simulink model "k1visetmymon"  (Simulink 8.6)
settings: Solver=VariableStepAuto  StartTime=0.0  StopTime=10.0  RelTol=1e-3
libraries: cdsIPCx x31, cdsFilt x2, cdsAdcx0 x1, cdsAdcx1 x1, cdsAdcx2 x1, VISMON_MASTER x1, cdsModelRate x1, cdsParameters x1
settings Model: Creator=controls  LastModifiedBy=controls
settings DataIOCC: SaveFormat=Dataset  SignalLoggingSaveFormat=Dataset
settings OptimizationCC: ExpressionDepthLimit=128
settings DebuggingCC: UnderspecifiedInitializationDetection=Simplified  MergeDetectMultiDrivingBlocksExec=error  SolverPrmCheckMsg=none  FcnCallInpInsideContextMsg=EnableAllAsError  StateNameClashWarn=none
settings HardwareCC: ProdBitPerPointer=64  ProdLargestAtomicFloat=Float  ProdIntDivRoundTo=Zero  ProdEndianess=LittleEndian  ProdWordSize=64  ProdHWDeviceType=Intel->x86-64 (Windows64)
settings GRTTargetCC: GeneratePreprocessorConditionals=Use local settings  CombineOutputUpdateFcns=on  GRTInterface=off
settings ConfigComp: CovModelRefEnable=off

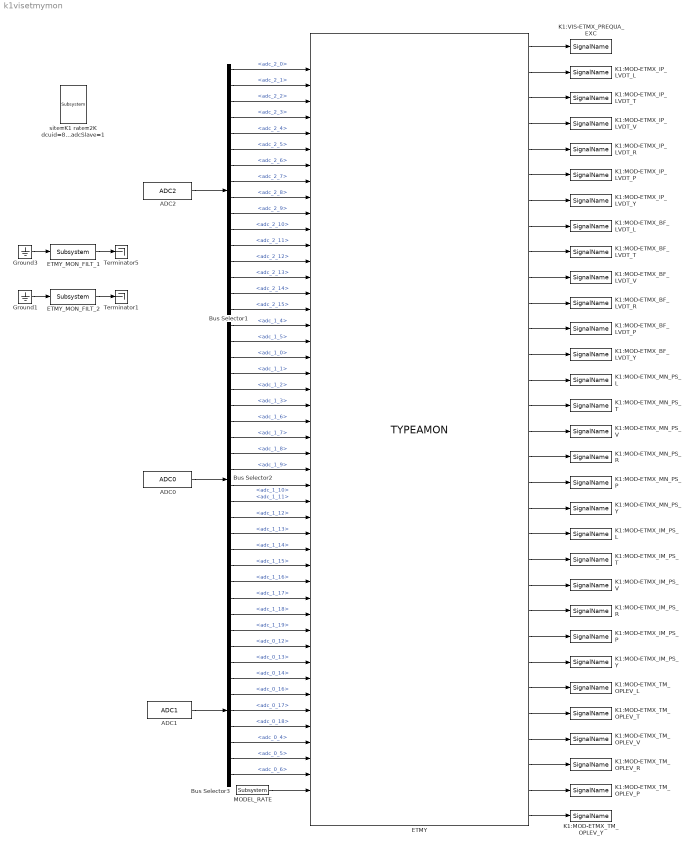
== system k1visetmymon ==
  ADC0 : cdsAdcx0/ADC0  Tag=cdsAdc  Description=|
      | type-GSC_16AI64SSA
      | card_num=0
      settings: AttributesFormatString=%<Description>\n%<Tag>
  ADC1 : cdsAdcx1/ADC1  Tag=cdsAdc  Description=|
      | type-GSC_16AI64SSA
      | card_num=1
      settings: AttributesFormatString=%<Description>\n%<Tag>
  ADC2 : cdsAdcx2/ADC2  Tag=cdsAdc  Description=|
      | type-GSC_16AI64SSA
      | card_num=2
      settings: AttributesFormatString=%<Description>\n%<Tag>
  Bus Selector1 : BusSelector  Description=ADC Selector  OutputSignals=adc_2_0,adc_2_1,adc_2_2,adc_2_3,adc_2_4,adc_2_5,adc_2_6,adc_2_7,adc_2_8,adc_2_9,adc_2_10,adc_2_11,adc_2_12,adc_2_13,adc_2_14,adc_2_15
      settings: AttributesFormatString=%<Description>
  Bus Selector2 : BusSelector  OutputSignals=adc_1_4,adc_1_5,adc_1_0,adc_1_1,adc_1_2,adc_1_3,adc_1_6,adc_1_7,adc_1_8,adc_1_9,adc_1_10,adc_1_11,adc_1_12,adc_1_13,adc_1_14,adc_1_15,adc_1_16,adc_1_17,adc_1_18,adc_1_19
  Bus Selector3 : BusSelector  OutputSignals=adc_0_12,adc_0_13,adc_0_14,adc_0_16,adc_0_17,adc_0_18,adc_0_4,adc_0_5,adc_0_6
  ETMY : VISMON_MASTER/TYPEAMON
  ETMY_MON_FILT_1 : cdsFilt/Subsystem  Tag=cdsFilt  Description=|
      | Purpose:                                                                                                                                                                                                                                  
      | Standard CDS IIR filter module.                                                                                                                                                                                                           
      |                                                                                                                                                                                                                                           
      | Operation:                                                                                                                                                                                                                                
      | Consists of 10 second order section IIR filters, plus a ramped gain stage. In FE code, also provides pre-defined test points and excitation channel inputs. The filter coefficients are defined in the LIGO system using the 'foton' tool.
      |                                                                                                                                                                                                                                           
      | Usage:                                                                                                                                                                                                                                    
      | Name the part with the desired filter module name.
      settings: AttributesFormatString=%<Tag>
  ETMY_MON_FILT_2 : cdsFilt/Subsystem  Tag=cdsFilt  Description=|
      | Purpose:                                                                                                                                                                                                                                  
      | Standard CDS IIR filter module.                                                                                                                                                                                                           
      |                                                                                                                                                                                                                                           
      | Operation:                                                                                                                                                                                                                                
      | Consists of 10 second order section IIR filters, plus a ramped gain stage. In FE code, also provides pre-defined test points and excitation channel inputs. The filter coefficients are defined in the LIGO system using the 'foton' tool.
      |                                                                                                                                                                                                                                           
      | Usage:                                                                                                                                                                                                                                    
      | Name the part with the desired filter module name.
      settings: AttributesFormatString=%<Tag>
  Ground1 : Ground
  Ground3 : Ground
  K1:MOD-ETMX_BF_LVDT_L : cdsIPCx/SignalName  Tag=cdsIPCx_SHMEM  Description=Inter-Process Communication via Shared memory.
      settings: AttributesFormatString=%<Tag>
  K1:MOD-ETMX_BF_LVDT_P : cdsIPCx/SignalName  Tag=cdsIPCx_SHMEM  Description=Inter-Process Communication via Shared memory.
      settings: AttributesFormatString=%<Tag>
  K1:MOD-ETMX_BF_LVDT_R : cdsIPCx/SignalName  Tag=cdsIPCx_SHMEM  Description=Inter-Process Communication via Shared memory.
      settings: AttributesFormatString=%<Tag>
  K1:MOD-ETMX_BF_LVDT_T : cdsIPCx/SignalName  Tag=cdsIPCx_SHMEM  Description=Inter-Process Communication via Shared memory.
      settings: AttributesFormatString=%<Tag>
  K1:MOD-ETMX_BF_LVDT_V : cdsIPCx/SignalName  Tag=cdsIPCx_SHMEM  Description=Inter-Process Communication via Shared memory.
      settings: AttributesFormatString=%<Tag>
  K1:MOD-ETMX_BF_LVDT_Y : cdsIPCx/SignalName  Tag=cdsIPCx_SHMEM  Description=Inter-Process Communication via Shared memory.
      settings: AttributesFormatString=%<Tag>
  K1:MOD-ETMX_IM_PS_L : cdsIPCx/SignalName  Tag=cdsIPCx_SHMEM  Description=Inter-Process Communication via Shared memory.
      settings: AttributesFormatString=%<Tag>
  K1:MOD-ETMX_IM_PS_P : cdsIPCx/SignalName  Tag=cdsIPCx_SHMEM  Description=Inter-Process Communication via Shared memory.
      settings: AttributesFormatString=%<Tag>
  K1:MOD-ETMX_IM_PS_R : cdsIPCx/SignalName  Tag=cdsIPCx_SHMEM  Description=Inter-Process Communication via Shared memory.
      settings: AttributesFormatString=%<Tag>
  K1:MOD-ETMX_IM_PS_T : cdsIPCx/SignalName  Tag=cdsIPCx_SHMEM  Description=Inter-Process Communication via Shared memory.
      settings: AttributesFormatString=%<Tag>
  K1:MOD-ETMX_IM_PS_V : cdsIPCx/SignalName  Tag=cdsIPCx_SHMEM  Description=Inter-Process Communication via Shared memory.
      settings: AttributesFormatString=%<Tag>
  K1:MOD-ETMX_IM_PS_Y : cdsIPCx/SignalName  Tag=cdsIPCx_SHMEM  Description=Inter-Process Communication via Shared memory.
      settings: AttributesFormatString=%<Tag>
  K1:MOD-ETMX_IP_LVDT_L : cdsIPCx/SignalName  Tag=cdsIPCx_SHMEM  Description=Inter-Process Communication via Shared memory.
      settings: AttributesFormatString=%<Tag>
  K1:MOD-ETMX_IP_LVDT_P : cdsIPCx/SignalName  Tag=cdsIPCx_SHMEM  Description=Inter-Process Communication via Shared memory.
      settings: AttributesFormatString=%<Tag>
  K1:MOD-ETMX_IP_LVDT_R : cdsIPCx/SignalName  Tag=cdsIPCx_SHMEM  Description=Inter-Process Communication via Shared memory.
      settings: AttributesFormatString=%<Tag>
  K1:MOD-ETMX_IP_LVDT_T : cdsIPCx/SignalName  Tag=cdsIPCx_SHMEM  Description=Inter-Process Communication via Shared memory.
      settings: AttributesFormatString=%<Tag>
  K1:MOD-ETMX_IP_LVDT_V : cdsIPCx/SignalName  Tag=cdsIPCx_SHMEM  Description=Inter-Process Communication via Shared memory.
      settings: AttributesFormatString=%<Tag>
  K1:MOD-ETMX_IP_LVDT_Y : cdsIPCx/SignalName  Tag=cdsIPCx_SHMEM  Description=Inter-Process Communication via Shared memory.
      settings: AttributesFormatString=%<Tag>
  K1:MOD-ETMX_MN_PS_L : cdsIPCx/SignalName  Tag=cdsIPCx_SHMEM  Description=Inter-Process Communication via Shared memory.
      settings: AttributesFormatString=%<Tag>
  K1:MOD-ETMX_MN_PS_P : cdsIPCx/SignalName  Tag=cdsIPCx_SHMEM  Description=Inter-Process Communication via Shared memory.
      settings: AttributesFormatString=%<Tag>
  K1:MOD-ETMX_MN_PS_R : cdsIPCx/SignalName  Tag=cdsIPCx_SHMEM  Description=Inter-Process Communication via Shared memory.
      settings: AttributesFormatString=%<Tag>
  K1:MOD-ETMX_MN_PS_T : cdsIPCx/SignalName  Tag=cdsIPCx_SHMEM  Description=Inter-Process Communication via Shared memory.
      settings: AttributesFormatString=%<Tag>
  K1:MOD-ETMX_MN_PS_V : cdsIPCx/SignalName  Tag=cdsIPCx_SHMEM  Description=Inter-Process Communication via Shared memory.
      settings: AttributesFormatString=%<Tag>
  K1:MOD-ETMX_MN_PS_Y : cdsIPCx/SignalName  Tag=cdsIPCx_SHMEM  Description=Inter-Process Communication via Shared memory.
      settings: AttributesFormatString=%<Tag>
  K1:MOD-ETMX_TM_OPLEV_L : cdsIPCx/SignalName  Tag=cdsIPCx_SHMEM  Description=Inter-Process Communication via Shared memory.
      settings: AttributesFormatString=%<Tag>
  K1:MOD-ETMX_TM_OPLEV_P : cdsIPCx/SignalName  Tag=cdsIPCx_SHMEM  Description=Inter-Process Communication via Shared memory.
      settings: AttributesFormatString=%<Tag>
  K1:MOD-ETMX_TM_OPLEV_R : cdsIPCx/SignalName  Tag=cdsIPCx_SHMEM  Description=Inter-Process Communication via Shared memory.
      settings: AttributesFormatString=%<Tag>
  K1:MOD-ETMX_TM_OPLEV_T : cdsIPCx/SignalName  Tag=cdsIPCx_SHMEM  Description=Inter-Process Communication via Shared memory.
      settings: AttributesFormatString=%<Tag>
  K1:MOD-ETMX_TM_OPLEV_V : cdsIPCx/SignalName  Tag=cdsIPCx_SHMEM  Description=Inter-Process Communication via Shared memory.
      settings: AttributesFormatString=%<Tag>
  K1:MOD-ETMX_TM_OPLEV_Y : cdsIPCx/SignalName  Tag=cdsIPCx_SHMEM  Description=Inter-Process Communication via Shared memory.
      settings: AttributesFormatString=%<Tag>
  K1:VIS-ETMX_PREQUA_EXC : cdsIPCx/SignalName  Tag=cdsIPCx_SHMEM  Description=Inter-Process Communication via Shared memory.
      settings: AttributesFormatString=%<Tag>
  MODEL_RATE : cdsModelRate/Subsystem  Tag=cdsModelRate
      settings: AttributesFormatString=%<Tag>
  Terminator1 : Terminator
  Terminator5 : Terminator
  site=K1 rate=2K dcuid=80 host=k1ey1 specific_cpu=1 adcSlave=1 : cdsParameters/Subsystem  Tag=cdsParameters  Description=|
      | Purpose:                                                                                                                                                                                                                                
      | Provide system parameters to the FE code generator to properly configure the generated EPICS names, rep rate of the FE controller, and the Data Acquisition node ID for proper storage of data from this FE controller.                 
      |                                                                                                                                                                                                                                         
      | Useage:                                                                                                                                                                                                                                 
      | The part NAME field is used to identify the FE parameters. It must be of the form:                                                                                                                                                      
      | site=                                                                                                                                                                                                                                   
      | rate=                                                                                                                                                                                                                                   
      | dcuid=                                                                                                                                                                                                                                  
      |                                                                                                                                                                                                                                         
      | Where:                                                                                                                                                                                                                                  
      | site= argument may be H1, H2, L1, M1, G1, either as a single argument or multiple, for example site=H1,H2. These are the only names allowed. These will become the first two characters of all EPICS and signal names (for example G1:).
      |                                                                                                                                                                                                                                         
      | rate= may be 2K, 16K, 32K, or 64K                                                                                                                                                                                                       
      |                                                                                                                                                                                                                                         
      | dcuid= is site specific ie it must be unique at each site.
      settings: AttributesFormatString=%<Tag>
  wires:
  ADC2/1 -> Bus Selector1/1
  Ground3/1 -> ETMY_MON_FILT_1/1
  Ground1/1 -> ETMY_MON_FILT_2/1
  ETMY_MON_FILT_1/1 -> Terminator5/1
  ETMY_MON_FILT_2/1 -> Terminator1/1
  Bus Selector1/1 -> ETMY/1  "<adc_2_0>"
  Bus Selector1/2 -> ETMY/2  "<adc_2_1>"
  Bus Selector1/3 -> ETMY/3  "<adc_2_2>"
  Bus Selector1/4 -> ETMY/4  "<adc_2_3>"
  Bus Selector1/5 -> ETMY/5  "<adc_2_4>"
  Bus Selector1/6 -> ETMY/6  "<adc_2_5>"
  Bus Selector1/7 -> ETMY/7  "<adc_2_6>"
  Bus Selector1/8 -> ETMY/8  "<adc_2_7>"
  Bus Selector1/9 -> ETMY/9  "<adc_2_8>"
  Bus Selector1/10 -> ETMY/10  "<adc_2_9>"
  Bus Selector1/11 -> ETMY/11  "<adc_2_10>"
  Bus Selector1/12 -> ETMY/12  "<adc_2_11>"
  Bus Selector1/13 -> ETMY/13  "<adc_2_12>"
  Bus Selector1/14 -> ETMY/14  "<adc_2_13>"
  Bus Selector1/15 -> ETMY/15  "<adc_2_14>"
  Bus Selector1/16 -> ETMY/16  "<adc_2_15>"
  Bus Selector2/2 -> ETMY/18  "<adc_1_5>"
  Bus Selector2/9 -> ETMY/25  "<adc_1_8>"
  Bus Selector2/3 -> ETMY/19  "<adc_1_0>"
  Bus Selector2/8 -> ETMY/24  "<adc_1_7>"
  Bus Selector2/13 -> ETMY/29  "<adc_1_12>"
  Bus Selector2/5 -> ETMY/21  "<adc_1_2>"
  Bus Selector2/14 -> ETMY/30  "<adc_1_13>"
  Bus Selector2/17 -> ETMY/33  "<adc_1_16>"
  Bus Selector2/12 -> ETMY/28  "<adc_1_11>"
  Bus Selector2/16 -> ETMY/32  "<adc_1_15>"
  Bus Selector2/20 -> ETMY/36  "<adc_1_19>"
  Bus Selector2/18 -> ETMY/34  "<adc_1_17>"
  Bus Selector2/11 -> ETMY/27  "<adc_1_10>"
  Bus Selector2/4 -> ETMY/20  "<adc_1_1>"
  Bus Selector2/6 -> ETMY/22  "<adc_1_3>"
  Bus Selector2/7 -> ETMY/23  "<adc_1_6>"
  Bus Selector2/1 -> ETMY/17  "<adc_1_4>"
  Bus Selector2/19 -> ETMY/35  "<adc_1_18>"
  Bus Selector2/15 -> ETMY/31  "<adc_1_14>"
  Bus Selector2/10 -> ETMY/26  "<adc_1_9>"
  Bus Selector3/2 -> ETMY/38  "<adc_0_13>"
  Bus Selector3/6 -> ETMY/42  "<adc_0_18>"
  Bus Selector3/1 -> ETMY/37  "<adc_0_12>"
  Bus Selector3/3 -> ETMY/39  "<adc_0_14>"
  Bus Selector3/5 -> ETMY/41  "<adc_0_17>"
  Bus Selector3/8 -> ETMY/44  "<adc_0_5>"
  Bus Selector3/7 -> ETMY/43  "<adc_0_4>"
  Bus Selector3/4 -> ETMY/40  "<adc_0_16>"
  Bus Selector3/9 -> ETMY/45  "<adc_0_6>"
  ADC1/1 -> Bus Selector3/1
  ADC0/1 -> Bus Selector2/1
  MODEL_RATE/1 -> ETMY/46
  ETMY/1 -> K1:VIS-ETMX_PREQUA_EXC/1
  ETMY/2 -> K1:MOD-ETMX_IP_LVDT_L/1
  ETMY/14 -> K1:MOD-ETMX_MN_PS_L/1
  ETMY/3 -> K1:MOD-ETMX_IP_LVDT_T/1
  ETMY/4 -> K1:MOD-ETMX_IP_LVDT_V/1
  ETMY/5 -> K1:MOD-ETMX_IP_LVDT_R/1
  ETMY/6 -> K1:MOD-ETMX_IP_LVDT_P/1
  ETMY/7 -> K1:MOD-ETMX_IP_LVDT_Y/1
  ETMY/8 -> K1:MOD-ETMX_BF_LVDT_L/1
  ETMY/9 -> K1:MOD-ETMX_BF_LVDT_T/1
  ETMY/10 -> K1:MOD-ETMX_BF_LVDT_V/1
  ETMY/11 -> K1:MOD-ETMX_BF_LVDT_R/1
  ETMY/12 -> K1:MOD-ETMX_BF_LVDT_P/1
  ETMY/13 -> K1:MOD-ETMX_BF_LVDT_Y/1
  ETMY/15 -> K1:MOD-ETMX_MN_PS_T/1
  ETMY/16 -> K1:MOD-ETMX_MN_PS_V/1
  ETMY/17 -> K1:MOD-ETMX_MN_PS_R/1
  ETMY/18 -> K1:MOD-ETMX_MN_PS_P/1
  ETMY/19 -> K1:MOD-ETMX_MN_PS_Y/1
  ETMY/20 -> K1:MOD-ETMX_IM_PS_L/1
  ETMY/21 -> K1:MOD-ETMX_IM_PS_T/1
  ETMY/22 -> K1:MOD-ETMX_IM_PS_V/1
  ETMY/23 -> K1:MOD-ETMX_IM_PS_R/1
  ETMY/24 -> K1:MOD-ETMX_IM_PS_P/1
  ETMY/25 -> K1:MOD-ETMX_IM_PS_Y/1
  ETMY/26 -> K1:MOD-ETMX_TM_OPLEV_L/1
  ETMY/27 -> K1:MOD-ETMX_TM_OPLEV_T/1
  ETMY/28 -> K1:MOD-ETMX_TM_OPLEV_V/1
  ETMY/29 -> K1:MOD-ETMX_TM_OPLEV_R/1
  ETMY/30 -> K1:MOD-ETMX_TM_OPLEV_P/1
  ETMY/31 -> K1:MOD-ETMX_TM_OPLEV_Y/1
